simulink model "six_bots_Observer_Collision_MN_VP_NAPF"  (R2021a)
settings: Solver=ode5  StartTime=0.0  StopTime=20  FixedStep=0.005  RelTol=1e-3
(part 3 of 4)

== matlab function six_bots_Observer_Collision_MN_VP_NAPF/Self Calculation 3/Topology changing and APF/Changing topology ==
  data: x_agents input; rel_distance output; L input; L_i output
function [rel_distance, L_i] = topology_update(x_agents, L)

%% Notes:
% The purpose of this function is to update the communication topology
% among agents according to their current locations
% position_agents: a (nN,1) vector to represent the current location of agents
% L: a (N,N) matrix to represent the fixed communication topology

%% Basic parameters

% Robot parameters
serial_num = 3;
R = 1.5; % predefined value of the limited range communication
dimension = 3;

% Time-varying topology parameter
eta_1 = 0.2;
eta_2 = 14; 
eta_3 = 1.1;


%% Useful information

num_agent = size(x_agents,1)/dimension;

rel_distance = zeros(num_agent,1);

cur_pos = x_agents( (serial_num-1)*dimension +1 :(serial_num-1)*dimension +2 );

L_i = L(serial_num,:);


%% Limited range communication

for i = 1:num_agent
   if i == serial_num
       rel_distance(i) = 0;
   else
       rel_vector = cur_pos - x_agents( (i-1)*dimension +1 :(i-1)*dimension +2 );
       rel_dis = sqrt(rel_vector'*rel_vector);
       
       if rel_dis <= R  % If the distance is close enough
           if L_i(i) > -1   % If there is no connection before
               L_i(i) = - eta_1*(1-1./(1+exp(-eta_2*(rel_dis-eta_3))));
               L_i(serial_num) = L_i(serial_num) - L_i(i);
           end
       end
       
       rel_distance(i) = rel_dis;
       
   end
    
end









end

== matlab function six_bots_Observer_Collision_MN_VP_NAPF/Self Calculation 3/Topology changing and APF/Communication based APF ==
  data: x_agents input; F_i output; L_i input
function F_i = commu_based_apf(x_agents, L_i)

%% Notes
% The purpose of this function is perform the APF based on known information

% L_i: a (1,N) vector that represents the communication among agents
% position_agents: the current position of agents

%% Basic parameters
serial_num = 3;
dimension = 3;

alpha = 2;
epsilon_1 = 1.1; % the parameter for the inner boundaries
epsilon_2 = 2; % the parameter for the outer boundaries

%% The info of current agent
Radius=[0.24;0.30;0.23;0.35;0.28;0.25];
r_i = Radius(serial_num);
pos_i = x_agents( (serial_num - 1)*dimension +1 : (serial_num - 1)*dimension +2 );
f_i = [0;0];

for j = 1 : size(L_i,2)
   if j == serial_num   % if it is the agent itself
       f_i = f_i + [0;0];
   else   % if not
       if L_i(j)<0  % if there are connections (meaning it is close enough)
           r_j = Radius(j);    % obtain the radius
           pos_j = x_agents( (j - 1)*dimension +1 : (j - 1)*dimension +2 );
           z_ij = pos_i - pos_j;
           r_in = epsilon_1 * (r_i + r_j);
           r_out = epsilon_2 * (r_i + r_j);
           if norm(z_ij) <= r_out      % if its within the range of APF
               f_ij = alpha* (r_out - norm(z_ij))/(norm(z_ij) - r_in)^2 * z_ij/norm(z_ij);
               f_i = f_i + f_ij;
           end
       end
   end
end

F_i = [f_i;0];
    




end

== matlab function six_bots_Observer_Collision_MN_VP_NAPF/Self Calculation 3/error calculation ==
  data: z input; delta_x output; reference_hat input; delta_v output; w_hat output; ad_hat output
function [delta_x, delta_v, w_hat, ad_hat] = error_calculation(z, reference_hat)

%% Notes
% The purpose of this function is to select and calculate useful information

dimension = 3;

x = z(dimension*0+1:dimension*1);
v_hat = z(dimension*1+1:dimension*2);
w_hat = z(dimension*2+1:dimension*3);

xd = reference_hat(dimension*0+1:dimension*1);
vd_hat = reference_hat(dimension*1+1:dimension*2);
ad_hat = reference_hat(dimension*2+1:dimension*3);

delta_x = x - xd;
delta_v = v_hat - vd_hat;



end

== matlab function six_bots_Observer_Collision_MN_VP_NAPF/Self Calculation 3/u_bar calculation ==
  data: F_i input; u_bar output; delta_x input; delta_v input; w_hat input; ad_hat input
function u_bar = u_bar_cal(F_i, delta_x, delta_v, w_hat, ad_hat)

%% This function aims to calculate a part of controller first

lambda = 2;

u_bar = -w_hat - lambda*delta_v - delta_x + ad_hat + F_i;



end

== matlab function six_bots_Observer_Collision_MN_VP_NAPF/Controller and Plant 5/Observation error 1 ==
  data: x input; v input; w input; ob_tilde output; Z input
function ob_tilde = estimation_error(x, v, w, Z)

% dimension=3;

state = [x;v;w];

ob_tilde = Z - state;

% x_hat = Z(dimension*0+1 :dimension*1);
% v_hat = Z(dimension*1+1 :dimension*2);
% w_hat = Z(dimension*2+1 :dimension*3);
% 
% x_tilde = x_hat - x;
% v_tilde = v_hat - v;
% w_tilde = w_hat - w; 



end

== matlab function six_bots_Observer_Collision_MN_VP_NAPF/Controller and Plant 4/SMC Controller ==
  data: pos input; u output; e_xi input; e_vi input; s output; u_bar input
function [u,s] = controller(pos, e_xi, e_vi, u_bar)

%% Note
% The function for the SMC controller 


%% basic data
Mass=[4.8;5.5;4.5;5.8;5.3;5.0];
Radius=[0.24;0.30;0.23;0.31;0.28;0.25];
Inertia=[0.15;0.25;0.12;0.29;0.21;0.15];

serial_num = 4;
dimension = 3; 

m=Mass(serial_num);
R=Radius(serial_num);
inertia=Inertia(serial_num);


%% parameters
lambda = 2;
c = 2;

s = e_vi + lambda* e_xi;

%% calculate g_bar
theta = pos(dimension);
M=diag([m,m,inertia]);
T=[-sin(theta), -sin(pi/3-theta), sin(pi/3+theta);
    cos(theta), -cos(pi/3-theta), -cos(pi/3+theta);
    R,          R,                  R];

g_bar = T^-1 * M;

u = g_bar * ( - c*s + u_bar);


end

== matlab function six_bots_Observer_Collision_MN_VP_NAPF/Controller and Plant 4/Select from communication ==
  data: info_commu input; e_xi output; L_i input; e_vi output
function [e_xi, e_vi] = commu_sele(info_commu, L_i)

%% Note

% The purpose of this function is to 
% 1) abstract the information for calculation
% 2) calculate local variables e_xi, e_vi

% The info_commu comes in the form of [delta_x; delta_v];

%% basic parameters
num_agent = size(L_i,2); 
dimension = 3;


%% abstract information from communication
abstract_x = kron(kron(eye(num_agent),[1,0]),eye(dimension));
abstract_v = kron(kron(eye(num_agent),[0,1]),eye(dimension));

delta_x = abstract_x * info_commu;
delta_v = abstract_v * info_commu;


e_xi = kron(L_i, eye(dimension) ) * delta_x;
e_vi = kron(L_i, eye(dimension) ) * delta_v;



end

== matlab function six_bots_Observer_Collision_MN_VP_NAPF/Self Calculation 1/u_bar calculation ==
  data: F_i input; u_bar output; delta_x input; delta_v input; w_hat input; ad_hat input
function u_bar = u_bar_cal(F_i, delta_x, delta_v, w_hat, ad_hat)

%% This function aims to calculate a part of controller first

lambda = 2;

u_bar = -w_hat - lambda*delta_v - delta_x + ad_hat + F_i;



end

== matlab function six_bots_Observer_Collision_MN_VP_NAPF/Controller and Plant 4/System Plant1 ==
  data: agent_x input; v_dot output; agent_v input; t input; control_input input; w output
function [v_dot, w] = physical_model( agent_x , agent_v, t, control_input )

%% Note
% System output
% v_dot: the acceleration vector
% w: the matched disturbances
% saturation status: off
% model is established by the driving force provided by the motor

%% basic parameters set of agents
Mass=[4.8;5.5;4.5;5.8;5.3;5.0];
Radius=[0.24;0.30;0.23;0.31;0.28;0.25];
Inertia=[0.15;0.25;0.12;0.29;0.21;0.15];

%% assign the parameter according to serial number
serial_num = 4; 
m=Mass(serial_num);
R=Radius(serial_num);
inertia=Inertia(serial_num);

%% current states of the robot
dimension=3;

x=agent_x(1);
y=agent_x(2);
theta=agent_x(dimension);

%% time-varying matched disturbances
% matched_disturbance= [0.5*sin(1.5*t+pi/4*serial_num+x)+2; 0.6*cos(2*t+pi/3*serial_num+0.5*y)+1.5; 0.5*sin(0.8*t+pi/5*serial_num+0.4*theta)+1];

% matched_disturbance= [0.5*sin(1.5*t+pi/4*serial_num)+2; 0.6*cos(2*t+pi/3*serial_num)+1.5; 0.5*sin(0.8*t+pi/5*serial_num)+1];

matched_disturbance = [0.5*sin(x) + tanh(x) + 0.6*sin(0.6*t + pi/5*serial_num); 0.3*sin(y) - 1.4*exp(-abs(y)-1) + 0.8*sin(0.4*t + pi/5*serial_num) ; 0.2 * cos(theta) + sin(0.5*t + pi/5*serial_num)];

%% the real model of robot
M=diag([1/m,1/m,1/inertia]);
T=[-sin(theta), -sin(pi/3-theta), sin(pi/3+theta);
    cos(theta), -cos(pi/3-theta), -cos(pi/3+theta);
    R,          R,                  R];

g=M*T;

%% plant output

w = matched_disturbance;

v_dot = w + g* control_input;


end

== matlab function six_bots_Observer_Collision_MN_VP_NAPF/Self Calculation 4/Neural network observer/Finite observer/Finite time observer/Initialisation/MATLAB Function ==
  data: t input; y output; x input
function y = initial(t,x)

if t==0
    y = [0;0;0];
else
    y = x;
end

end

== matlab function six_bots_Observer_Collision_MN_VP_NAPF/Self Calculation 4/Neural network observer/Finite observer/Finite time observer/Observer ==
  data: f_hat input; z input; u input; x input; z_dot output; x_tilde output
function [z_dot, x_tilde] = observer(f_hat, z, u, x)

dimension = 3;

%% Substracting information from observation

z_1 = z(dimension*0+1:dimension*1);
z_2 = z(dimension*1+1:dimension*2);

x_tilde = z_1 - x;

%% basic parameters set of agents
Mass=[4.8;5.5;4.5;5.8;5.3;5.0];
Radius=[0.24;0.30;0.23;0.31;0.28;0.25];
Inertia=[0.15;0.25;0.12;0.29;0.21;0.15];

%% assign the parameter according to serial number
serial_num = 4; 
m=Mass(serial_num);
R=Radius(serial_num);
inertia=Inertia(serial_num);
theta = x(dimension);

%% the real model of robot
M=diag([1/m,1/m,1/inertia]);
T=[-sin(theta), -sin(pi/3-theta), sin(pi/3+theta);
    cos(theta), -cos(pi/3-theta), -cos(pi/3+theta);
    R,          R,                  R];
g=M*T;

%% Parameters

beta_1 = 2/3;
beta_2 = 2 * beta_1 - 1;

alpha_1 = 8;
alpha_2 = 8;


z_1_dot = z_2 - alpha_1 * sign(x_tilde) .* abs(x_tilde).^beta_1;
z_2_dot = - alpha_2 * sign(x_tilde) .* abs(x_tilde).^beta_2 + g * u + f_hat;


z_dot = [z_1_dot; z_2_dot];

end

== matlab function six_bots_Observer_Collision_MN_VP_NAPF/Self Calculation 4/Neural network observer/Finite observer/Neural network/MATLAB Function ==
  data: x_tilde output; phi output; z input; W input; x input; w_dot output; b output; k output
function [ x_tilde, phi, w_dot, b, k] = weight_update(z, W, x)

%% This function aims to update the neural network weights inside the observer
% z =[z_1;z_2] is a 6*1 matrix
% phi_nn represents the input is a g*1 matrix (depends on different nn used)
% W represents the weight is a 3*g matrix (depends on different nn used)
% Here, g=6

%% substracting information
dimension = 3;

x_hat = z(dimension*0+1:dimension*1);
v_hat = z(dimension*1+1:dimension*2);

x_tilde = x_hat - x;

%% Parameter of the observer
beta_1 = 2/3;
c = sign(x_tilde).*abs(x_tilde).^beta_1;
b = norm(c);


%% Input of the neural network

% Try multiple entries of RBF neural network

% Wideth of Gaussian function
mu = 8;

% Number of middle layer nurons
n_num = 8;
phi = zeros(n_num,1);

% The input vector of RBFNN
y_i = [x ; v_hat];

% Calculate each nuron in the middle layer
for j = 1 : n_num
    
   % Centre of the receptive field
   % Method 1: unified values (Result: bounded within 0.0045)
   d_j = (j-3) * ones(2 * dimension, 1);
   
   % Method 2: varying centre (Result: bounded within 0.0535 Conclusion: not working)
%    d_j = 1-dimension : 1 : dimension;
%    d_j = (j-3) * d_j';
   
   phi_j = exp(-(y_i - d_j)'*(y_i - d_j)/mu^2); 
    
   phi(j) = phi_j;
end







%% Static parameter
% k_1 = -20000;
% k_2 = -1000;

% k_1 = -5000;
% k_2 = -500;

%% Varying parameters
if b>=1
    k_1 = -1;
    k_2 = -0.05;
elseif b<1 && b>=10^(-1) 
    k_1 = -5;
    k_2 = -0.25;
elseif b<10^(-1) && b>=10^(-2)
    k_1 = -50;
    k_2 = -5;
elseif b<10^(-2) && b>=10^(-3)
    k_1 = -200;
    k_2 = -20;
else
    k_1 = -10000;
    k_2 = -100;    
% elseif b<10^(-3) && b>=10^(-4)
%     k_1 = -5000;
%     k_2 = -30;
% else
%     k_1 = -10000;
%     k_2 = -100;
end

k = [k_1;k_2];

w_dot = k_1 * ( c * phi' ) + k_2 * b * W ; 

% A different way to design the update rate (WORKS)
% w_dot = k_1 * ( phi_nn * x_tilde) ; 



end

== matlab function six_bots_Observer_Collision_MN_VP_NAPF/Self Calculation 4/Neural network observer/Finite observer/Neural network/NN approximation ==
  data: phi_nn input; W input; f_hat output
function f_hat = nn_approximation(phi_nn, W)

%% Neural network approximation
% f_hat = W^T * phi_nn
% phi_nn = [x,v_hat]^T



f_hat = W * phi_nn;

end

== matlab function six_bots_Observer_Collision_MN_VP_NAPF/Self Calculation 4/Neural network observer/Finite observer/Neural network/NN initialisation ==
  data: W_in output
function W_in = nn_initial()

dimension = 3;
n_num = 8;

W_in= zeros(dimension,n_num);

end

== matlab function six_bots_Observer_Collision_MN_VP_NAPF/Self Calculation 4/Neural network observer/Finite observer/Select useful information ==
  data: f_hat input; z input; z_new output; x input; z_used output
function [z_new, z_used] = fcn(f_hat, z, x)

dimension = 3;

z_new = [z ; f_hat];
z_used = [x; z(dimension*1+1:dimension*2) ; f_hat];

end

== matlab function six_bots_Observer_Collision_MN_VP_NAPF/Self Calculation 4/Neural network observer/Position selection ==
  data: x_agents input; x_agent output
function x_agent = pos_selection(x_agents)

%% Notes
% This function aims to select the current agent's position information

dimension = 3;
serial_num = 4;

x_agent = x_agents ( (serial_num - 1)*dimension+1 : serial_num*dimension );


end

== matlab function six_bots_Observer_Collision_MN_VP_NAPF/Self Calculation 4/Sliding mode differentiator/MATLAB Function ==
  data: z input; x_d input; esti_references output
function esti_references = pack_n_send(z, x_d)

dimension = 3;

esti_references = [x_d;z(dimension*1+1:dimension*3)];



end

== matlab function six_bots_Observer_Collision_MN_VP_NAPF/Self Calculation 4/Sliding mode differentiator/Reference selection ==
  data: reference input; agent_reference output
function agent_reference = reference_select(reference)

%% Notes
% The purpose of this function is to select the position reference for
% the current agent

serial_num = 4;
dimension = 3;


agent_reference = reference ( (serial_num - 1)*dimension + 1 : serial_num*dimension );



end

== matlab function six_bots_Observer_Collision_MN_VP_NAPF/Self Calculation 4/Sliding mode differentiator/sliding mode differentiator ==
  data: z input; z_dot output; x_d input
function z_dot = sliding_diff(z,x_d)

%% This is the observer function that estimates the unknown reference derivatives

dimension = 3;

alpha_1 = 6;
alpha_2 = 8;
alpha_3 = 8;
alpha_4 = 6;

beta_xd = 0.1;

xi_1 = z(dimension*0+1:dimension*1);
xi_2 = z(dimension*1+1:dimension*2);
xi_3 = z(dimension*2+1:dimension*3);
xi_4 = z(dimension*3+1:dimension*4);

%% tunning
nu_1 = -alpha_1 * power(beta_xd,1/4) * power(abs(xi_1-x_d),3/4) .* sign(xi_1-x_d) + xi_2;
nu_2 = -alpha_2 * power(beta_xd,1/3) * power(abs(xi_2-nu_1),2/3) .* sign(xi_2-nu_1) +xi_3;
nu_3 = -alpha_3 * power(beta_xd,1/2) * power(abs(xi_3-nu_2),1/2) .* sign(xi_3-nu_2) +xi_4;
nu_4 = -alpha_4 * beta_xd .* sign(xi_4-nu_3);

z_dot = [nu_1;nu_2;nu_3;nu_4];


end

== matlab function six_bots_Observer_Collision_MN_VP_NAPF/Self Calculation 4/Topology changing and APF/Changing topology ==
  data: x_agents input; rel_distance output; L input; L_i output
function [rel_distance, L_i] = topology_update(x_agents, L)

%% Notes:
% The purpose of this function is to update the communication topology
% among agents according to their current locations
% position_agents: a (nN,1) vector to represent the current location of agents
% L: a (N,N) matrix to represent the fixed communication topology

%% Basic parameters

% Robot parameters
serial_num = 4;
R = 1.5; % predefined value of the limited range communication
dimension = 3;

% Time-varying topology parameter
eta_1 = 0.2;
eta_2 = 14; 
eta_3 = 1.1;


%% Useful information

num_agent = size(x_agents,1)/dimension;

rel_distance = zeros(num_agent,1);

cur_pos = x_agents( (serial_num-1)*dimension +1 :(serial_num-1)*dimension +2 );

L_i = L(serial_num,:);


%% Limited range communication

for i = 1:num_agent
   if i == serial_num
       rel_distance(i) = 0;
   else
       rel_vector = cur_pos - x_agents( (i-1)*dimension +1 :(i-1)*dimension +2 );
       rel_dis = sqrt(rel_vector'*rel_vector);
       
       if rel_dis <= R  % If the distance is close enough
           if L_i(i) > -1   % If there is no connection before
               L_i(i) = - eta_1*(1-1./(1+exp(-eta_2*(rel_dis-eta_3))));
               L_i(serial_num) = L_i(serial_num) - L_i(i);
           end
       end
       
       rel_distance(i) = rel_dis;
       
   end
    
end









end

== matlab function six_bots_Observer_Collision_MN_VP_NAPF/Self Calculation 4/Topology changing and APF/Communication based APF ==
  data: x_agents input; F_i output; L_i input
function F_i = commu_based_apf(x_agents, L_i)

%% Notes
% The purpose of this function is perform the APF based on known information

% L_i: a (1,N) vector that represents the communication among agents
% position_agents: the current position of agents

%% Basic parameters
serial_num = 4;
dimension = 3;

alpha = 2;
epsilon_1 = 1.1; % the parameter for the inner boundaries
epsilon_2 = 2; % the parameter for the outer boundaries

%% The info of current agent
Radius=[0.24;0.30;0.23;0.31;0.28;0.25];
r_i = Radius(serial_num);
pos_i = x_agents( (serial_num - 1)*dimension +1 : (serial_num - 1)*dimension +2 );
f_i = [0;0];

for j = 1 : size(L_i,2)
   if j == serial_num   % if it is the agent itself
       f_i = f_i + [0;0];
   else   % if not
       if L_i(j)<0  % if there are connections (meaning it is close enough)
           r_j = Radius(j);    % obtain the radius
           pos_j = x_agents( (j - 1)*dimension +1 : (j - 1)*dimension +2 );
           z_ij = pos_i - pos_j;
           r_in = epsilon_1 * (r_i + r_j);
           r_out = epsilon_2 * (r_i + r_j);
           if norm(z_ij) <= r_out      % if its within the range of APF
               f_ij = alpha* (r_out - norm(z_ij))/(norm(z_ij) - r_in)^2 * z_ij/norm(z_ij);
               f_i = f_i + f_ij;
           end
       end
   end
end

F_i = [f_i;0];
    




end

== matlab function six_bots_Observer_Collision_MN_VP_NAPF/Self Calculation 1/Neural network observer/Finite observer/Finite time observer/Observer ==
  data: f_hat input; z input; u input; x input; z_dot output; x_tilde output
function [z_dot, x_tilde] = observer(f_hat, z, u, x)

dimension = 3;

%% Substracting information from observation

z_1 = z(dimension*0+1:dimension*1);
z_2 = z(dimension*1+1:dimension*2);

x_tilde = z_1 - x;

%% basic parameters set of agents
Mass=[4.8;5.5;4.5;5.8;5.3;5.0];
Radius=[0.24;0.30;0.23;0.35;0.28;0.25];
Inertia=[0.15;0.25;0.12;0.35;0.21;0.15];

%% assign the parameter according to serial number
serial_num = 1; 
m=Mass(serial_num);
R=Radius(serial_num);
inertia=Inertia(serial_num);
theta = x(dimension);

%% the real model of robot
M=diag([1/m,1/m,1/inertia]);
T=[-sin(theta), -sin(pi/3-theta), sin(pi/3+theta);
    cos(theta), -cos(pi/3-theta), -cos(pi/3+theta);
    R,          R,                  R];
g=M*T;

%% Parameters

beta_1 = 2/3;
beta_2 = 2 * beta_1 - 1;

alpha_1 = 8;
alpha_2 = 8;


z_1_dot = z_2 - alpha_1 * sign(x_tilde) .* abs(x_tilde).^beta_1;
z_2_dot = - alpha_2 * sign(x_tilde) .* abs(x_tilde).^beta_2 + g * u + f_hat;


z_dot = [z_1_dot; z_2_dot];

end

== matlab function six_bots_Observer_Collision_MN_VP_NAPF/Self Calculation 4/error calculation ==
  data: z input; delta_x output; reference_hat input; delta_v output; w_hat output; ad_hat output
function [delta_x, delta_v, w_hat, ad_hat] = error_calculation(z, reference_hat)

%% Notes
% The purpose of this function is to select and calculate useful information

dimension = 3;

x = z(dimension*0+1:dimension*1);
v_hat = z(dimension*1+1:dimension*2);
w_hat = z(dimension*2+1:dimension*3);

xd = reference_hat(dimension*0+1:dimension*1);
vd_hat = reference_hat(dimension*1+1:dimension*2);
ad_hat = reference_hat(dimension*2+1:dimension*3);

delta_x = x - xd;
delta_v = v_hat - vd_hat;



end

== matlab function six_bots_Observer_Collision_MN_VP_NAPF/Self Calculation 4/u_bar calculation ==
  data: F_i input; u_bar output; delta_x input; delta_v input; w_hat input; ad_hat input
function u_bar = u_bar_cal(F_i, delta_x, delta_v, w_hat, ad_hat)

%% This function aims to calculate a part of controller first

lambda = 2;

u_bar = -w_hat - lambda*delta_v - delta_x + ad_hat + F_i;



end

== matlab function six_bots_Observer_Collision_MN_VP_NAPF/Controller and Plant 6/Observation error 1 ==
  data: x input; v input; w input; ob_tilde output; Z input
function ob_tilde = estimation_error(x, v, w, Z)

% dimension=3;

state = [x;v;w];

ob_tilde = Z - state;

% x_hat = Z(dimension*0+1 :dimension*1);
% v_hat = Z(dimension*1+1 :dimension*2);
% w_hat = Z(dimension*2+1 :dimension*3);
% 
% x_tilde = x_hat - x;
% v_tilde = v_hat - v;
% w_tilde = w_hat - w; 



end

== matlab function six_bots_Observer_Collision_MN_VP_NAPF/Controller and Plant 5/SMC Controller ==
  data: pos input; u output; e_xi input; e_vi input; s output; u_bar input
function [u,s] = controller(pos, e_xi, e_vi, u_bar)

%% Note
% The function for the SMC controller 


%% basic data
Mass=[4.8;5.5;4.5;5.8;5.3;5.0];
Radius=[0.24;0.30;0.23;0.35;0.28;0.25];
Inertia=[0.15;0.25;0.12;0.35;0.21;0.15];

serial_num = 5;
dimension = 3; 

m=Mass(serial_num);
R=Radius(serial_num);
inertia=Inertia(serial_num);


%% parameters
lambda = 2;
c = 2;

s = e_vi + lambda* e_xi;

%% calculate g_bar
theta = pos(dimension);
M=diag([m,m,inertia]);
T=[-sin(theta), -sin(pi/3-theta), sin(pi/3+theta);
    cos(theta), -cos(pi/3-theta), -cos(pi/3+theta);
    R,          R,                  R];

g_bar = T^-1 * M;

u = g_bar * ( - c*s + u_bar);


end

== matlab function six_bots_Observer_Collision_MN_VP_NAPF/Controller and Plant 5/Select from communication ==
  data: info_commu input; e_xi output; L_i input; e_vi output
function [e_xi, e_vi] = commu_sele(info_commu, L_i)

%% Note

% The purpose of this function is to 
% 1) abstract the information for calculation
% 2) calculate local variables e_xi, e_vi

% The info_commu comes in the form of [delta_x; delta_v];

%% basic parameters
num_agent = size(L_i,2); 
dimension = 3;


%% abstract information from communication
abstract_x = kron(kron(eye(num_agent),[1,0]),eye(dimension));
abstract_v = kron(kron(eye(num_agent),[0,1]),eye(dimension));

delta_x = abstract_x * info_commu;
delta_v = abstract_v * info_commu;


e_xi = kron(L_i, eye(dimension) ) * delta_x;
e_vi = kron(L_i, eye(dimension) ) * delta_v;



end

== matlab function six_bots_Observer_Collision_MN_VP_NAPF/Controller and Plant 5/System Plant1 ==
  data: agent_x input; v_dot output; agent_v input; t input; control_input input; w output
function [v_dot, w] = physical_model( agent_x , agent_v, t, control_input )

%% Note
% System output
% v_dot: the acceleration vector
% w: the matched disturbances
% saturation status: off
% model is established by the driving force provided by the motor

%% basic parameters set of agents
Mass=[4.8;5.5;4.5;5.8;5.3;5.0];
Radius=[0.24;0.30;0.23;0.31;0.28;0.25];
Inertia=[0.15;0.25;0.12;0.29;0.21;0.15];

%% assign the parameter according to serial number
serial_num = 5; 
m=Mass(serial_num);
R=Radius(serial_num);
inertia=Inertia(serial_num);

%% current states of the robot
dimension=3;

x=agent_x(1);
y=agent_x(2);
theta=agent_x(dimension);

%% time-varying matched disturbances
% matched_disturbance= [0.5*sin(1.5*t+pi/4*serial_num+x)+2; 0.6*cos(2*t+pi/3*serial_num+0.5*y)+1.5; 0.5*sin(0.8*t+pi/5*serial_num+0.4*theta)+1];

% matched_disturbance= [0.5*sin(1.5*t+pi/4*serial_num)+2; 0.6*cos(2*t+pi/3*serial_num)+1.5; 0.5*sin(0.8*t+pi/5*serial_num)+1];

matched_disturbance = [0.5*sin(x) + tanh(x) + 0.6*sin(0.6*t + pi/5*serial_num); 0.3*sin(y) - 1.4*exp(-abs(y)-1) + 0.8*sin(0.4*t + pi/5*serial_num) ; 0.2 * cos(theta) + sin(0.5*t + pi/5*serial_num)];

%% the real model of robot
M=diag([1/m,1/m,1/inertia]);
T=[-sin(theta), -sin(pi/3-theta), sin(pi/3+theta);
    cos(theta), -cos(pi/3-theta), -cos(pi/3+theta);
    R,          R,                  R];

g=M*T;

%% plant output

w = matched_disturbance;

v_dot = w + g* control_input;


end

== matlab function six_bots_Observer_Collision_MN_VP_NAPF/Self Calculation 5/Neural network observer/Finite observer/Finite time observer/Initialisation/MATLAB Function ==
  data: t input; y output; x input
function y = initial(t,x)

if t==0
    y = [0;0;0];
else
    y = x;
end

end

== matlab function six_bots_Observer_Collision_MN_VP_NAPF/Self Calculation 5/Neural network observer/Finite observer/Finite time observer/Observer ==
  data: f_hat input; z input; u input; x input; z_dot output; x_tilde output
function [z_dot, x_tilde] = observer(f_hat, z, u, x)

dimension = 3;

%% Substracting information from observation

z_1 = z(dimension*0+1:dimension*1);
z_2 = z(dimension*1+1:dimension*2);

x_tilde = z_1 - x;

%% basic parameters set of agents
Mass=[4.8;5.5;4.5;5.8;5.3;5.0];
Radius=[0.24;0.30;0.23;0.35;0.28;0.25];
Inertia=[0.15;0.25;0.12;0.35;0.21;0.15];

%% assign the parameter according to serial number
serial_num = 5; 
m=Mass(serial_num);
R=Radius(serial_num);
inertia=Inertia(serial_num);
theta = x(dimension);

%% the real model of robot
M=diag([1/m,1/m,1/inertia]);
T=[-sin(theta), -sin(pi/3-theta), sin(pi/3+theta);
    cos(theta), -cos(pi/3-theta), -cos(pi/3+theta);
    R,          R,                  R];
g=M*T;

%% Parameters

beta_1 = 2/3;
beta_2 = 2 * beta_1 - 1;

alpha_1 = 8;
alpha_2 = 8;


z_1_dot = z_2 - alpha_1 * sign(x_tilde) .* abs(x_tilde).^beta_1;
z_2_dot = - alpha_2 * sign(x_tilde) .* abs(x_tilde).^beta_2 + g * u + f_hat;


z_dot = [z_1_dot; z_2_dot];

end

== matlab function six_bots_Observer_Collision_MN_VP_NAPF/Self Calculation 5/Neural network observer/Finite observer/Neural network/MATLAB Function ==
  data: x_tilde output; phi output; z input; W input; x input; w_dot output; b output; k output
function [ x_tilde, phi, w_dot, b, k] = weight_update(z, W, x)

%% This function aims to update the neural network weights inside the observer
% z =[z_1;z_2] is a 6*1 matrix
% phi_nn represents the input is a g*1 matrix (depends on different nn used)
% W represents the weight is a 3*g matrix (depends on different nn used)
% Here, g=6

%% substracting information
dimension = 3;

x_hat = z(dimension*0+1:dimension*1);
v_hat = z(dimension*1+1:dimension*2);

x_tilde = x_hat - x;

%% Parameter of the observer
beta_1 = 2/3;
c = sign(x_tilde).*abs(x_tilde).^beta_1;
b = norm(c);


%% Input of the neural network

% Try multiple entries of RBF neural network

% Wideth of Gaussian function
mu = 8;

% Number of middle layer nurons
n_num = 8;
phi = zeros(n_num,1);

% The input vector of RBFNN
y_i = [x ; v_hat];

% Calculate each nuron in the middle layer
for j = 1 : n_num
    
   % Centre of the receptive field
   % Method 1: unified values (Result: bounded within 0.0045)
   d_j = (j-3) * ones(2 * dimension, 1);
   
   % Method 2: varying centre (Result: bounded within 0.0535 Conclusion: not working)
%    d_j = 1-dimension : 1 : dimension;
%    d_j = (j-3) * d_j';
   
   phi_j = exp(-(y_i - d_j)'*(y_i - d_j)/mu^2); 
    
   phi(j) = phi_j;
end







%% Static parameter
% k_1 = -20000;
% k_2 = -1000;

% k_1 = -5000;
% k_2 = -500;

%% Varying parameters
if b>=1
    k_1 = -1;
    k_2 = -0.05;
elseif b<1 && b>=10^(-1) 
    k_1 = -5;
    k_2 = -0.25;
elseif b<10^(-1) && b>=10^(-2)
    k_1 = -50;
    k_2 = -5;
elseif b<10^(-2) && b>=10^(-3)
    k_1 = -200;
    k_2 = -20;
else
    k_1 = -10000;
    k_2 = -100;    
% elseif b<10^(-3) && b>=10^(-4)
%     k_1 = -5000;
%     k_2 = -30;
% else
%     k_1 = -10000;
%     k_2 = -100;
end

k = [k_1;k_2];

w_dot = k_1 * ( c * phi' ) + k_2 * b * W ; 

% A different way to design the update rate (WORKS)
% w_dot = k_1 * ( phi_nn * x_tilde) ; 



end

== matlab function six_bots_Observer_Collision_MN_VP_NAPF/Self Calculation 5/Neural network observer/Finite observer/Neural network/NN approximation ==
  data: phi_nn input; W input; f_hat output
function f_hat = nn_approximation(phi_nn, W)

%% Neural network approximation
% f_hat = W^T * phi_nn
% phi_nn = [x,v_hat]^T



f_hat = W * phi_nn;

end

== matlab function six_bots_Observer_Collision_MN_VP_NAPF/Self Calculation 1/Neural network observer/Finite observer/Select useful information ==
  data: f_hat input; z input; z_new output; x input; z_used output
function [z_new, z_used] = fcn(f_hat, z, x)

dimension = 3;

z_new = [z ; f_hat];
z_used = [x; z(dimension*1+1:dimension*2) ; f_hat];

end

== matlab function six_bots_Observer_Collision_MN_VP_NAPF/Self Calculation 5/Neural network observer/Finite observer/Neural network/NN initialisation ==
  data: W_in output
function W_in = nn_initial()

dimension = 3;
n_num = 8;

W_in= zeros(dimension,n_num);

end

== matlab function six_bots_Observer_Collision_MN_VP_NAPF/Self Calculation 5/Neural network observer/Finite observer/Select useful information ==
  data: f_hat input; z input; z_new output; x input; z_used output
function [z_new, z_used] = fcn(f_hat, z, x)

dimension = 3;

z_new = [z ; f_hat];
z_used = [x; z(dimension*1+1:dimension*2) ; f_hat];

end

== matlab function six_bots_Observer_Collision_MN_VP_NAPF/Self Calculation 5/Neural network observer/Position selection ==
  data: x_agents input; x_agent output
function x_agent = pos_selection(x_agents)

%% Notes
% This function aims to select the current agent's position information

dimension = 3;
serial_num = 5;

x_agent = x_agents ( (serial_num - 1)*dimension+1 : serial_num*dimension );


end

== matlab function six_bots_Observer_Collision_MN_VP_NAPF/Self Calculation 5/Sliding mode differentiator/MATLAB Function ==
  data: z input; x_d input; esti_references output
function esti_references = pack_n_send(z, x_d)

dimension = 3;

esti_references = [x_d;z(dimension*1+1:dimension*3)];



end

== matlab function six_bots_Observer_Collision_MN_VP_NAPF/Self Calculation 5/Sliding mode differentiator/Reference selection ==
  data: reference input; agent_reference output
function agent_reference = reference_select(reference)

%% Notes
% The purpose of this function is to select the position reference for
% the current agent

serial_num = 5;
dimension = 3;


agent_reference = reference ( (serial_num - 1)*dimension + 1 : serial_num*dimension );



end

== matlab function six_bots_Observer_Collision_MN_VP_NAPF/Self Calculation 5/Sliding mode differentiator/sliding mode differentiator ==
  data: z input; z_dot output; x_d input
function z_dot = sliding_diff(z,x_d)

%% This is the observer function that estimates the unknown reference derivatives

dimension = 3;

alpha_1 = 6;
alpha_2 = 8;
alpha_3 = 8;
alpha_4 = 6;

beta_xd = 0.1;

xi_1 = z(dimension*0+1:dimension*1);
xi_2 = z(dimension*1+1:dimension*2);
xi_3 = z(dimension*2+1:dimension*3);
xi_4 = z(dimension*3+1:dimension*4);

%% tunning
nu_1 = -alpha_1 * power(beta_xd,1/4) * power(abs(xi_1-x_d),3/4) .* sign(xi_1-x_d) + xi_2;
nu_2 = -alpha_2 * power(beta_xd,1/3) * power(abs(xi_2-nu_1),2/3) .* sign(xi_2-nu_1) +xi_3;
nu_3 = -alpha_3 * power(beta_xd,1/2) * power(abs(xi_3-nu_2),1/2) .* sign(xi_3-nu_2) +xi_4;
nu_4 = -alpha_4 * beta_xd .* sign(xi_4-nu_3);

z_dot = [nu_1;nu_2;nu_3;nu_4];


end

== matlab function six_bots_Observer_Collision_MN_VP_NAPF/Self Calculation 5/Topology changing and APF/Changing topology ==
  data: x_agents input; rel_distance output; L input; L_i output
function [rel_distance, L_i] = topology_update(x_agents, L)

%% Notes:
% The purpose of this function is to update the communication topology
% among agents according to their current locations
% position_agents: a (nN,1) vector to represent the current location of agents
% L: a (N,N) matrix to represent the fixed communication topology

%% Basic parameters

% Robot parameters
serial_num = 5;
R = 1.5; % predefined value of the limited range communication
dimension = 3;

% Time-varying topology parameter
eta_1 = 0.2;
eta_2 = 14; 
eta_3 = 1.1;


%% Useful information

num_agent = size(x_agents,1)/dimension;

rel_distance = zeros(num_agent,1);

cur_pos = x_agents( (serial_num-1)*dimension +1 :(serial_num-1)*dimension +2 );

L_i = L(serial_num,:);


%% Limited range communication

for i = 1:num_agent
   if i == serial_num
       rel_distance(i) = 0;
   else
       rel_vector = cur_pos - x_agents( (i-1)*dimension +1 :(i-1)*dimension +2 );
       rel_dis = sqrt(rel_vector'*rel_vector);
       
       if rel_dis <= R  % If the distance is close enough
           if L_i(i) > -1   % If there is no connection before
               L_i(i) = - eta_1*(1-1./(1+exp(-eta_2*(rel_dis-eta_3))));
               L_i(serial_num) = L_i(serial_num) - L_i(i);
           end
       end
       
       rel_distance(i) = rel_dis;
       
   end
    
end









end

== matlab function six_bots_Observer_Collision_MN_VP_NAPF/Self Calculation 5/Topology changing and APF/Communication based APF ==
  data: x_agents input; F_i output; L_i input
function F_i = commu_based_apf(x_agents, L_i)

%% Notes
% The purpose of this function is perform the APF based on known information

% L_i: a (1,N) vector that represents the communication among agents
% position_agents: the current position of agents

%% Basic parameters
serial_num = 5;
dimension = 3;

alpha = 2;
epsilon_1 = 1.1; % the parameter for the inner boundaries
epsilon_2 = 2; % the parameter for the outer boundaries

%% The info of current agent
Radius=[0.24;0.30;0.23;0.35;0.28;0.25];
r_i = Radius(serial_num);
pos_i = x_agents( (serial_num - 1)*dimension +1 : (serial_num - 1)*dimension +2 );
f_i = [0;0];

for j = 1 : size(L_i,2)
   if j == serial_num   % if it is the agent itself
       f_i = f_i + [0;0];
   else   % if not
       if L_i(j)<0  % if there are connections (meaning it is close enough)
           r_j = Radius(j);    % obtain the radius
           pos_j = x_agents( (j - 1)*dimension +1 : (j - 1)*dimension +2 );
           z_ij = pos_i - pos_j;
           r_in = epsilon_1 * (r_i + r_j);
           r_out = epsilon_2 * (r_i + r_j);
           if norm(z_ij) <= r_out      % if its within the range of APF
               f_ij = alpha* (r_out - norm(z_ij))/(norm(z_ij) - r_in)^2 * z_ij/norm(z_ij);
               f_i = f_i + f_ij;
           end
       end
   end
end

F_i = [f_i;0];
    




end

== matlab function six_bots_Observer_Collision_MN_VP_NAPF/Self Calculation 5/error calculation ==
  data: z input; delta_x output; reference_hat input; delta_v output; w_hat output; ad_hat output
function [delta_x, delta_v, w_hat, ad_hat] = error_calculation(z, reference_hat)

%% Notes
% The purpose of this function is to select and calculate useful information

dimension = 3;

x = z(dimension*0+1:dimension*1);
v_hat = z(dimension*1+1:dimension*2);
w_hat = z(dimension*2+1:dimension*3);

xd = reference_hat(dimension*0+1:dimension*1);
vd_hat = reference_hat(dimension*1+1:dimension*2);
ad_hat = reference_hat(dimension*2+1:dimension*3);

delta_x = x - xd;
delta_v = v_hat - vd_hat;



end

== matlab function six_bots_Observer_Collision_MN_VP_NAPF/Self Calculation 5/u_bar calculation ==
  data: F_i input; u_bar output; delta_x input; delta_v input; w_hat input; ad_hat input
function u_bar = u_bar_cal(F_i, delta_x, delta_v, w_hat, ad_hat)

%% This function aims to calculate a part of controller first

lambda = 2;

u_bar = -w_hat - lambda*delta_v - delta_x + ad_hat + F_i;



end

== matlab function six_bots_Observer_Collision_MN_VP_NAPF/ob_data_processing ==
  data: ob_tilde_1 input; norm_tilde output; ob_tilde_2 input; ob_tilde_3 input; ob_tilde_4 input; ob_tilde_5 input; ob_tilde_6 input
function norm_tilde = ob_data(ob_tilde_1,ob_tilde_2, ob_tilde_3, ob_tilde_4, ob_tilde_5, ob_tilde_6)


norm_x = norm(ob_tilde_1(1:3)) + norm(ob_tilde_2(1:3)) + norm(ob_tilde_3(1:3)) + norm(ob_tilde_4(1:3)) + norm(ob_tilde_5(1:3)) + norm(ob_tilde_6(1:3));
norm_y = norm(ob_tilde_1(4:6)) + norm(ob_tilde_2(4:6)) + norm(ob_tilde_3(4:6)) + norm(ob_tilde_4(4:6)) + norm(ob_tilde_5(4:6)) + norm(ob_tilde_6(4:6));
norm_w = norm(ob_tilde_1(7:9)) + norm(ob_tilde_2(7:9)) + norm(ob_tilde_3(7:9)) + norm(ob_tilde_4(7:9)) + norm(ob_tilde_5(7:9)) + norm(ob_tilde_6(7:9));

norm_tilde = [norm_x; norm_y; norm_w]; 






end

== matlab function six_bots_Observer_Collision_MN_VP_NAPF/Controller and Plant 6/SMC Controller ==
  data: pos input; u output; e_xi input; e_vi input; s output; u_bar input
function [u,s] = controller(pos, e_xi, e_vi, u_bar)

%% Note
% The function for the SMC controller 


%% basic data
Mass=[4.8;5.5;4.5;5.8;5.3;5.0];
Radius=[0.24;0.30;0.23;0.35;0.28;0.25];
Inertia=[0.15;0.25;0.12;0.35;0.21;0.15];

serial_num = 6;
dimension = 3; 

m=Mass(serial_num);
R=Radius(serial_num);
inertia=Inertia(serial_num);


%% parameters
lambda = 2;
c = 2;

s = e_vi + lambda* e_xi;

%% calculate g_bar
theta = pos(dimension);
M=diag([m,m,inertia]);
T=[-sin(theta), -sin(pi/3-theta), sin(pi/3+theta);
    cos(theta), -cos(pi/3-theta), -cos(pi/3+theta);
    R,          R,                  R];

g_bar = T^-1 * M;

u = g_bar * ( - c*s + u_bar);


end

== matlab function six_bots_Observer_Collision_MN_VP_NAPF/Controller and Plant 2/Select from communication ==
  data: info_commu input; e_xi output; L_i input; e_vi output
function [e_xi, e_vi] = commu_sele(info_commu, L_i)

%% Note

% The purpose of this function is to 
% 1) abstract the information for calculation
% 2) calculate local variables e_xi, e_vi

% The info_commu comes in the form of [delta_x; delta_v];

%% basic parameters
num_agent = size(L_i,2); 
dimension = 3;


%% abstract information from communication
abstract_x = kron(kron(eye(num_agent),[1,0]),eye(dimension));
abstract_v = kron(kron(eye(num_agent),[0,1]),eye(dimension));

delta_x = abstract_x * info_commu;
delta_v = abstract_v * info_commu;


e_xi = kron(L_i, eye(dimension) ) * delta_x;
e_vi = kron(L_i, eye(dimension) ) * delta_v;



end

== matlab function six_bots_Observer_Collision_MN_VP_NAPF/Controller and Plant 6/Select from communication ==
  data: info_commu input; e_xi output; L_i input; e_vi output
function [e_xi, e_vi] = commu_sele(info_commu, L_i)

%% Note

% The purpose of this function is to 
% 1) abstract the information for calculation
% 2) calculate local variables e_xi, e_vi

% The info_commu comes in the form of [delta_x; delta_v];

%% basic parameters
num_agent = size(L_i,2); 
dimension = 3;


%% abstract information from communication
abstract_x = kron(kron(eye(num_agent),[1,0]),eye(dimension));
abstract_v = kron(kron(eye(num_agent),[0,1]),eye(dimension));

delta_x = abstract_x * info_commu;
delta_v = abstract_v * info_commu;


e_xi = kron(L_i, eye(dimension) ) * delta_x;
e_vi = kron(L_i, eye(dimension) ) * delta_v;



end

== matlab function six_bots_Observer_Collision_MN_VP_NAPF/Controller and Plant 6/System Plant1 ==
  data: agent_x input; v_dot output; agent_v input; t input; control_input input; w output
function [v_dot, w] = physical_model( agent_x , agent_v, t, control_input )

%% Note
% System output
% v_dot: the acceleration vector
% w: the matched disturbances
% saturation status: off
% model is established by the driving force provided by the motor

%% basic parameters set of agents
Mass=[4.8;5.5;4.5;5.8;5.3;5.0];
Radius=[0.24;0.30;0.23;0.31;0.28;0.25];
Inertia=[0.15;0.25;0.12;0.29;0.21;0.15];

%% assign the parameter according to serial number
serial_num = 6; 
m=Mass(serial_num);
R=Radius(serial_num);
inertia=Inertia(serial_num);

%% current states of the robot
dimension=3;

x=agent_x(1);
y=agent_x(2);
theta=agent_x(dimension);

%% time-varying matched disturbances
% matched_disturbance= [0.5*sin(1.5*t+pi/4*serial_num+x)+2; 0.6*cos(2*t+pi/3*serial_num+0.5*y)+1.5; 0.5*sin(0.8*t+pi/5*serial_num+0.4*theta)+1];

% matched_disturbance= [0.5*sin(1.5*t+pi/4*serial_num)+2; 0.6*cos(2*t+pi/3*serial_num)+1.5; 0.5*sin(0.8*t+pi/5*serial_num)+1];

matched_disturbance = [0.5*sin(x) + tanh(x) + 0.6*sin(0.6*t + pi/5*serial_num); 0.3*sin(y) - 1.4*exp(-abs(y)-1) + 0.8*sin(0.4*t + pi/5*serial_num) ; 0.2 * cos(theta) + sin(0.5*t + pi/5*serial_num)];

%% the real model of robot
M=diag([1/m,1/m,1/inertia]);
T=[-sin(theta), -sin(pi/3-theta), sin(pi/3+theta);
    cos(theta), -cos(pi/3-theta), -cos(pi/3+theta);
    R,          R,                  R];

g=M*T;

%% plant output

w = matched_disturbance;

v_dot = w + g* control_input;


end

== matlab function six_bots_Observer_Collision_MN_VP_NAPF/Self Calculation 6/Neural network observer/Finite observer/Finite time observer/Initialisation/MATLAB Function ==
  data: t input; y output; x input
function y = initial(t,x)

if t==0
    y = [0;0;0];
else
    y = x;
end

end

== matlab function six_bots_Observer_Collision_MN_VP_NAPF/Self Calculation 6/Neural network observer/Finite observer/Finite time observer/Observer ==
  data: f_hat input; z input; u input; x input; z_dot output; x_tilde output
function [z_dot, x_tilde] = observer(f_hat, z, u, x)

dimension = 3;

%% Substracting information from observation

z_1 = z(dimension*0+1:dimension*1);
z_2 = z(dimension*1+1:dimension*2);

x_tilde = z_1 - x;

%% basic parameters set of agents
Mass=[4.8;5.5;4.5;5.8;5.3;5.0];
Radius=[0.24;0.30;0.23;0.35;0.28;0.25];
Inertia=[0.15;0.25;0.12;0.35;0.21;0.15];

%% assign the parameter according to serial number
serial_num = 3; 
m=Mass(serial_num);
R=Radius(serial_num);
inertia=Inertia(serial_num);
theta = x(dimension);

%% the real model of robot
M=diag([1/m,1/m,1/inertia]);
T=[-sin(theta), -sin(pi/3-theta), sin(pi/3+theta);
    cos(theta), -cos(pi/3-theta), -cos(pi/3+theta);
    R,          R,                  R];
g=M*T;

%% Parameters

beta_1 = 2/3;
beta_2 = 2 * beta_1 - 1;

alpha_1 = 8;
alpha_2 = 8;


z_1_dot = z_2 - alpha_1 * sign(x_tilde) .* abs(x_tilde).^beta_1;
z_2_dot = - alpha_2 * sign(x_tilde) .* abs(x_tilde).^beta_2 + g * u + f_hat;


z_dot = [z_1_dot; z_2_dot];

end

== matlab function six_bots_Observer_Collision_MN_VP_NAPF/Self Calculation 6/Neural network observer/Finite observer/Neural network/MATLAB Function ==
  data: x_tilde output; phi output; z input; W input; x input; w_dot output; b output; k output
function [ x_tilde, phi, w_dot, b, k] = weight_update(z, W, x)

%% This function aims to update the neural network weights inside the observer
% z =[z_1;z_2] is a 6*1 matrix
% phi_nn represents the input is a g*1 matrix (depends on different nn used)
% W represents the weight is a 3*g matrix (depends on different nn used)
% Here, g=6

%% substracting information
dimension = 3;

x_hat = z(dimension*0+1:dimension*1);
v_hat = z(dimension*1+1:dimension*2);

x_tilde = x_hat - x;

%% Parameter of the observer
beta_1 = 2/3;
c = sign(x_tilde).*abs(x_tilde).^beta_1;
b = norm(c);


%% Input of the neural network

% Try multiple entries of RBF neural network

% Wideth of Gaussian function
mu = 8;

% Number of middle layer nurons
n_num = 8;
phi = zeros(n_num,1);

% The input vector of RBFNN
y_i = [x ; v_hat];

% Calculate each nuron in the middle layer
for j = 1 : n_num
    
   % Centre of the receptive field
   % Method 1: unified values (Result: bounded within 0.0045)
   d_j = (j-3) * ones(2 * dimension, 1);
   
   % Method 2: varying centre (Result: bounded within 0.0535 Conclusion: not working)
%    d_j = 1-dimension : 1 : dimension;
%    d_j = (j-3) * d_j';
   
   phi_j = exp(-(y_i - d_j)'*(y_i - d_j)/mu^2); 
    
   phi(j) = phi_j;
end







%% Static parameter
% k_1 = -20000;
% k_2 = -1000;

% k_1 = -5000;
% k_2 = -500;

%% Varying parameters
if b>=1
    k_1 = -1;
    k_2 = -0.05;
elseif b<1 && b>=10^(-1) 
    k_1 = -5;
    k_2 = -0.25;
elseif b<10^(-1) && b>=10^(-2)
    k_1 = -50;
    k_2 = -5;
elseif b<10^(-2) && b>=10^(-3)
    k_1 = -200;
    k_2 = -20;
else
    k_1 = -10000;
    k_2 = -100;    
% elseif b<10^(-3) && b>=10^(-4)
%     k_1 = -5000;
%     k_2 = -30;
% else
%     k_1 = -10000;
%     k_2 = -100;
end

k = [k_1;k_2];

w_dot = k_1 * ( c * phi' ) + k_2 * b * W ; 

% A different way to design the update rate (WORKS)
% w_dot = k_1 * ( phi_nn * x_tilde) ; 



end

== matlab function six_bots_Observer_Collision_MN_VP_NAPF/Self Calculation 6/Neural network observer/Finite observer/Neural network/NN approximation ==
  data: phi_nn input; W input; f_hat output
function f_hat = nn_approximation(phi_nn, W)

%% Neural network approximation
% f_hat = W^T * phi_nn
% phi_nn = [x,v_hat]^T



f_hat = W * phi_nn;

end

== matlab function six_bots_Observer_Collision_MN_VP_NAPF/Self Calculation 6/Neural network observer/Finite observer/Neural network/NN initialisation ==
  data: W_in output
function W_in = nn_initial()

dimension = 3;
n_num = 8;

W_in= zeros(dimension,n_num);

end

== matlab function six_bots_Observer_Collision_MN_VP_NAPF/Self Calculation 6/Neural network observer/Finite observer/Select useful information ==
  data: f_hat input; z input; z_new output; x input; z_used output
function [z_new, z_used] = fcn(f_hat, z, x)

dimension = 3;

z_new = [z ; f_hat];
z_used = [x; z(dimension*1+1:dimension*2) ; f_hat];

end

== matlab function six_bots_Observer_Collision_MN_VP_NAPF/Self Calculation 6/Neural network observer/Position selection ==
  data: x_agents input; x_agent output
function x_agent = pos_selection(x_agents)

%% Notes
% This function aims to select the current agent's position information

dimension = 3;
serial_num = 6;

x_agent = x_agents ( (serial_num - 1)*dimension+1 : serial_num*dimension );


end

== matlab function six_bots_Observer_Collision_MN_VP_NAPF/Controller and Plant 1/SMC Controller ==
  data: pos input; u output; e_xi input; e_vi input; s output; u_bar input
function [u,s] = controller(pos, e_xi, e_vi, u_bar)

%% Note
% The function for the SMC controller 


%% basic data
Mass=[4.8;5.5;4.5;5.8;5.3;5.0];
Radius=[0.24;0.30;0.23;0.35;0.28;0.25];
Inertia=[0.15;0.25;0.12;0.35;0.21;0.15];

serial_num = 1;
dimension = 3; 

m=Mass(serial_num);
R=Radius(serial_num);
inertia=Inertia(serial_num);


%% parameters
lambda = 2;
c = 2;

s = e_vi + lambda* e_xi;

%% calculate g_bar
theta = pos(dimension);
M=diag([m,m,inertia]);
T=[-sin(theta), -sin(pi/3-theta), sin(pi/3+theta);
    cos(theta), -cos(pi/3-theta), -cos(pi/3+theta);
    R,          R,                  R];

g_bar = T^-1 * M;

u = g_bar * ( - c*s + u_bar);


end

== matlab function six_bots_Observer_Collision_MN_VP_NAPF/Self Calculation 6/Sliding mode differentiator/MATLAB Function ==
  data: z input; x_d input; esti_references output
function esti_references = pack_n_send(z, x_d)

dimension = 3;

esti_references = [x_d;z(dimension*1+1:dimension*3)];



end

== matlab function six_bots_Observer_Collision_MN_VP_NAPF/Self Calculation 6/Sliding mode differentiator/Reference selection ==
  data: reference input; agent_reference output
function agent_reference = reference_select(reference)

%% Notes
% The purpose of this function is to select the position reference for
% the current agent

serial_num = 6;
dimension = 3;


agent_reference = reference ( (serial_num - 1)*dimension + 1 : serial_num*dimension );



end

== matlab function six_bots_Observer_Collision_MN_VP_NAPF/Self Calculation 6/Sliding mode differentiator/sliding mode differentiator ==
  data: z input; z_dot output; x_d input
function z_dot = sliding_diff(z,x_d)

%% This is the observer function that estimates the unknown reference derivatives

dimension = 3;

alpha_1 = 6;
alpha_2 = 8;
alpha_3 = 8;
alpha_4 = 6;

beta_xd = 0.1;

xi_1 = z(dimension*0+1:dimension*1);
xi_2 = z(dimension*1+1:dimension*2);
xi_3 = z(dimension*2+1:dimension*3);
xi_4 = z(dimension*3+1:dimension*4);

%% tunning
nu_1 = -alpha_1 * power(beta_xd,1/4) * power(abs(xi_1-x_d),3/4) .* sign(xi_1-x_d) + xi_2;
nu_2 = -alpha_2 * power(beta_xd,1/3) * power(abs(xi_2-nu_1),2/3) .* sign(xi_2-nu_1) +xi_3;
nu_3 = -alpha_3 * power(beta_xd,1/2) * power(abs(xi_3-nu_2),1/2) .* sign(xi_3-nu_2) +xi_4;
nu_4 = -alpha_4 * beta_xd .* sign(xi_4-nu_3);

z_dot = [nu_1;nu_2;nu_3;nu_4];


end

== matlab function six_bots_Observer_Collision_MN_VP_NAPF/Self Calculation 6/Topology changing and APF/Changing topology ==
  data: x_agents input; rel_distance output; L input; L_i output
function [rel_distance, L_i] = topology_update(x_agents, L)

%% Notes:
% The purpose of this function is to update the communication topology
% among agents according to their current locations
% position_agents: a (nN,1) vector to represent the current location of agents
% L: a (N,N) matrix to represent the fixed communication topology

%% Basic parameters

% Robot parameters
serial_num = 6;
R = 1.5; % predefined value of the limited range communication
dimension = 3;

% Time-varying topology parameter
eta_1 = 0.2;
eta_2 = 14; 
eta_3 = 1.1;


%% Useful information

num_agent = size(x_agents,1)/dimension;

rel_distance = zeros(num_agent,1);

cur_pos = x_agents( (serial_num-1)*dimension +1 :(serial_num-1)*dimension +2 );

L_i = L(serial_num,:);


%% Limited range communication

for i = 1:num_agent
   if i == serial_num
       rel_distance(i) = 0;
   else
       rel_vector = cur_pos - x_agents( (i-1)*dimension +1 :(i-1)*dimension +2 );
       rel_dis = sqrt(rel_vector'*rel_vector);
       
       if rel_dis <= R  % If the distance is close enough
           if L_i(i) > -1   % If there is no connection before
               L_i(i) = - eta_1*(1-1./(1+exp(-eta_2*(rel_dis-eta_3))));
               L_i(serial_num) = L_i(serial_num) - L_i(i);
           end
       end
       
       rel_distance(i) = rel_dis;
       
   end
    
end









end
